simulink model "ABS_System"  (R2020b)
settings: Solver=VariableStepAuto  StartTime=0.0  StopTime=25  RelTol=1e-3
values from neighbouring files (symbols this model uses):
  g = 9.81    [Variables.m]
  I = 5    [Variables.m]
  m = 75    [Variables.m]
  R = 1.25    [Variables.m]
  v0 = 44    [Variables.m]
settings Model: Creator=samar  LastModifiedBy=samar
settings DataIOCC: SaveOutput=off  SaveTime=off

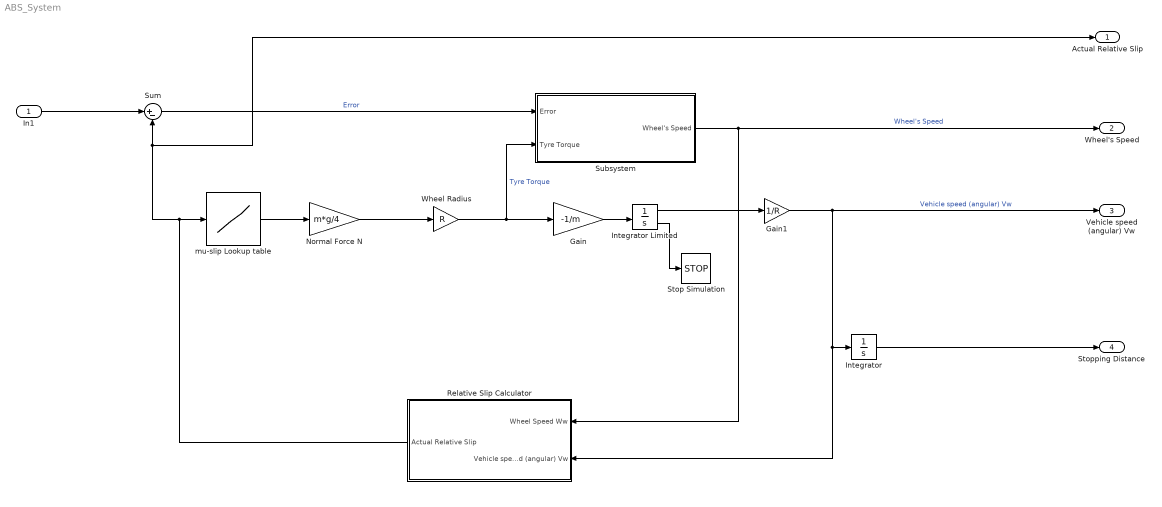
== system ABS_System ==
  In1 : Inport  OutDataTypeStr=double  PortDimensions=1
  Gain : Gain  Gain=-1/m
  Gain1 : Gain  Gain=1/R
  Integrator : Integrator
  Integrator Limited : Integrator  InitialCondition=v0  LimitOutput=on  UpperSaturationLimit=1000  LowerSaturationLimit=0  ShowSaturationPort=on
  Normal Force N : Gain  Gain=m*g/4
  Relative Slip Calculator : Subsystem
  Stop Simulation : Stop
  Subsystem : Subsystem
  Sum : Sum  Inputs=|+-
  Wheel Radius : Gain  Gain=R
  mu-slip Lookup table : Lookup_n-D  NumberOfTableDimensions=1  BreakpointsForDimension1=[0,0.05,0.1,0.15,0.2,0.25,0.3,0.35,0.4,0.45,0.5,0.55,0.6,0.65,0.7,0.75,0.8,0.85,0.9,0.95,1]  Table=[0,0.4,0.8,0.97,1,0.98,0.96,0.94,0.92,0.9,0.88,0.855,0.83,0.81,0.79,0.77,0.75,0.73,0.72,0.71,0.7]  InternalRulePriority=Speed  RndMeth=Simplest  InputSameDT=on
  Actual Relative Slip : Outport  OutDataTypeStr=double  PortDimensions=1  SampleTime=0
  Wheel's Speed : Outport  Port=2  OutDataTypeStr=double  PortDimensions=1  SampleTime=0
  Vehicle speed (angular) Vw : Outport  Port=3  OutDataTypeStr=double  PortDimensions=1  SampleTime=0
  Stopping Distance : Outport  Port=4  OutDataTypeStr=double  PortDimensions=1  SampleTime=0
  wires:
  Normal Force N/1 -> Wheel Radius/1
  Integrator Limited/1 -> Gain1/1
  Wheel Radius/1 -> Subsystem/2(Tyre Torque), Gain/1  "Tyre Torque"
  Gain1/1 -> Relative Slip Calculator/2(Vehicle speed (angular) Vw), Integrator/1, Vehicle speed (angular) Vw/1  "Vehicle speed (angular) Vw"
  Subsystem/1(Wheel's Speed) -> Wheel's Speed/1, Relative Slip Calculator/1(Wheel Speed Ww)  "Wheel's Speed"
  mu-slip Lookup table/1 -> Normal Force N/1
  Sum/1 -> Subsystem/1(Error)  "Error"
  Relative Slip Calculator/1(Actual Relative Slip) -> mu-slip Lookup table/1, Sum/2, Actual Relative Slip/1
  Gain/1 -> Integrator Limited/1
  Integrator Limited/2 -> Stop Simulation/1
  Integrator/1 -> Stopping Distance/1
  In1/1 -> Sum/1

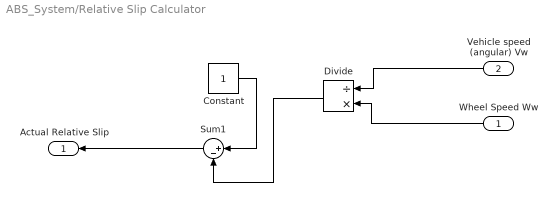
== system ABS_System/Relative Slip Calculator ==
  Wheel Speed Ww : Inport
  Vehicle speed (angular) Vw : Inport  Port=2
  Constant : Constant
  Divide : Product  Inputs=/*
  Sum1 : Sum  Inputs=|+-
  Actual Relative Slip : Outport
  wires:
  Vehicle speed (angular) Vw/1 -> Divide/1
  Divide/1 -> Sum1/2
  Wheel Speed Ww/1 -> Divide/2
  Constant/1 -> Sum1/1
  Sum1/1 -> Actual Relative Slip/1

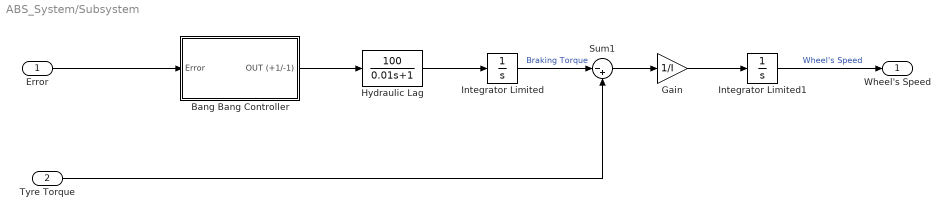
== system ABS_System/Subsystem ==
  Error : Inport
  Tyre Torque : Inport  Port=2
  Bang Bang Controller : Subsystem
  Gain : Gain  Gain=1/I
  Hydraulic Lag : TransferFcn  Numerator=[100]  Denominator=[0.01 1]
  Integrator Limited : Integrator  LimitOutput=on  UpperSaturationLimit=1000  LowerSaturationLimit=0
  Integrator Limited1 : Integrator  InitialCondition=v0/R  LimitOutput=on  UpperSaturationLimit=1000  LowerSaturationLimit=0
  Sum1 : Sum  Inputs=|-+
  Wheel's Speed : Outport
  wires:
  Integrator Limited1/1 -> Wheel's Speed/1  "Wheel's Speed"
  Gain/1 -> Integrator Limited1/1
  Tyre Torque/1 -> Sum1/2
  Sum1/1 -> Gain/1
  Integrator Limited/1 -> Sum1/1  "Braking Torque"
  Error/1 -> Bang Bang Controller/1(Error)
  Bang Bang Controller/1(OUT (+1/-1)) -> Hydraulic Lag/1
  Hydraulic Lag/1 -> Integrator Limited/1

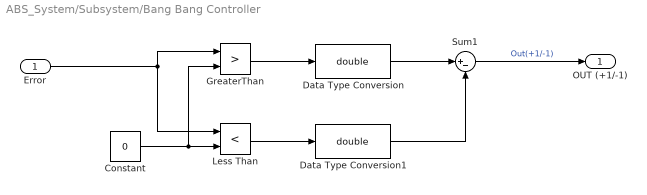
== system ABS_System/Subsystem/Bang Bang Controller ==
  Error : Inport
  Constant : Constant  Value=0
  Data Type Conversion : DataTypeConversion  OutDataTypeStr=double  RndMeth=Zero
  Data Type Conversion1 : DataTypeConversion  OutDataTypeStr=double  RndMeth=Zero
  GreaterThan : RelationalOperator  Operator=>  OutDataTypeStr=boolean  RndMeth=Simplest
  Less Than : RelationalOperator  Operator=<  OutDataTypeStr=boolean  RndMeth=Simplest
  Sum1 : Sum  Inputs=|+-
  OUT (+1/-1) : Outport
  wires:
  Data Type Conversion1/1 -> Sum1/2
  Error/1 -> Less Than/1, GreaterThan/1
  Sum1/1 -> OUT (+1/-1)/1  "Out(+1/-1)"
  GreaterThan/1 -> Data Type Conversion/1
  Data Type Conversion/1 -> Sum1/1
  Less Than/1 -> Data Type Conversion1/1
  Constant/1 -> Less Than/2, GreaterThan/2
